simulink model "vehicle_simulation"  (R2020a)
settings: Solver=ode1  StartTime=0.0  StopTime=500  FixedStep=0.1  RelTol=1e-3
undefined symbols (not defined in the file): HDBK, MIL, serial
libraries: powerlib_meascontrol x7, aerolibconvert2 x5, aerolibatmos2 x3, instrumentlib x3, dspsrcs4 x2, simulink x1
(part 5 of 5)

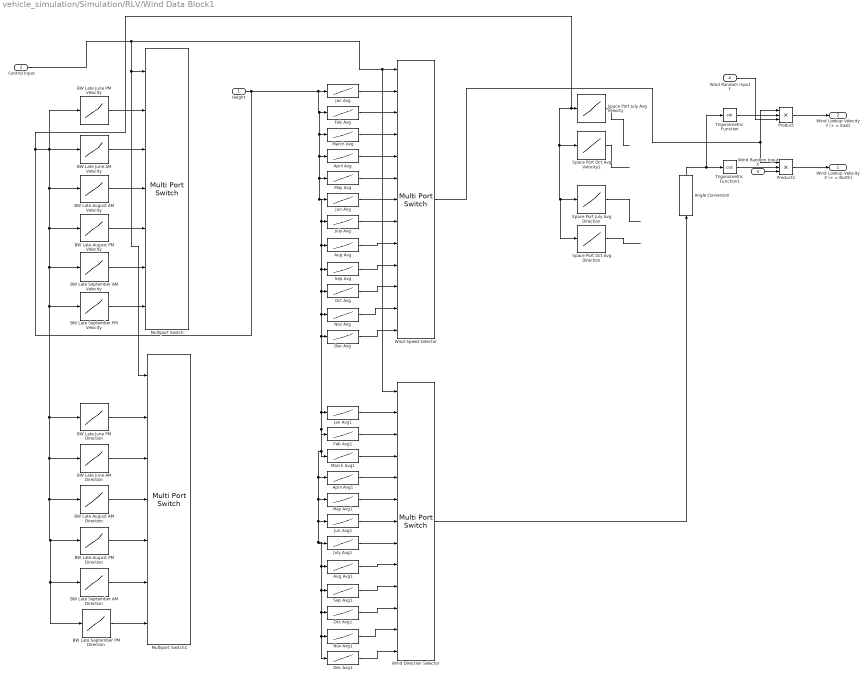
== system vehicle_simulation/Simulation/RLV/Wind Data Block1 ==
  Height : Inport
  Control Input : Inport  Port=2
  Wind Random Input X : Inport  Port=3
  Wind Random Input Y : Inport  Port=4
  Angle Conversion : aerolibconvert2/Angle Conversion  IU=deg  OU=rad
  April Avg : Lookup_n-D  NumberOfTableDimensions=1  BreakpointsForDimension1=[0,5000,10000,15000,20000,24000,100000]  Table=[5,17,30,20,5,7,0]  ExtrapMethod=Clip  UseLastTableValue=on  InternalRulePriority=Speed  RndMeth=Simplest  InputSameDT=on
  April Avg1 : Lookup_n-D  NumberOfTableDimensions=1  BreakpointsForDimension1=[0,5000,10000,15000,20000,24000,100000]  Table=[76,81,82,78,76,69,69]  ExtrapMethod=Clip  UseLastTableValue=on  InternalRulePriority=Speed  RndMeth=Simplest  InputSameDT=on
  Aug Avg : Lookup_n-D  NumberOfTableDimensions=1  BreakpointsForDimension1=[0,5000,10000,15000,20000,24000,100000]  Table=[2,2,5,2,10,14,0]  ExtrapMethod=Clip  UseLastTableValue=on  InternalRulePriority=Speed  RndMeth=Simplest  InputSameDT=on
  Aug Avg1 : Lookup_n-D  NumberOfTableDimensions=1  BreakpointsForDimension1=[0,5000,10000,15000,20000,24000,100000]  Table=[4,289,63,315,273,275,275]  ExtrapMethod=Clip  UseLastTableValue=on  InternalRulePriority=Speed  RndMeth=Simplest  InputSameDT=on
  BW Late August AM Direction : Lookup_n-D  NumberOfTableDimensions=1  BreakpointsForDimension1=[1546.1,1672.3,1845.1,2022.5,2255.5,2513.3,2836.4,3141.1,3395.8,3721.8,4061.2,4331.2,4582.8,4769.4,4942.4,5153.1,5313.9,5529.6,5694.8,5886,6078.5,6266.6,6490.2,6681.6,6882.9,7107.7,7346.2,7560,7827.5,8089.4,8305.8,8552.6,8781.9,9076.5,9311.2,9617.9,9889.3,10128,10375.7,10665.3,10948,11296.3,11552.9,11850.8,12069.6,12365.4,12654,12923.3,13134.5,13346.7,13598.6,13830.3,14097.1,14348,14557.6,14784.6,15036.1,15280.6,15487.7,15749.3,16059.5,16283.4,16572.3,16811.6,17109.6,17372.4,17652.2,17851.6,18135.9,18444.7,18704.6,19006.8,19282,19550.5,19765,20080.7,20374.9,20691.4,21007,21208.3,21458.2,21730.5,22033.2,22269.7,22494.3,22499.6,22744.1,22960,23248.2,23450.9,23683.3,23936.4,24175.2,24392.6,24677.4,24921.7,25201.5,25500,25741.8,25981.6,26271.3,26550.1,26831.4,27099.6,27393,27493.8,27652.2,27741,28143.9,28217,28571.1,28767.7,28789.4,29086.3,29225.3,29399.3,29535.7,29920.3,30157.2,30251.3,30403.5,30734,31253,31646,31990.8,32148.3,32309,32417,32931,80000]  Table=[228.9,227.3,225.3,226.4,224.6,219.5,200.9,219,197.3,198.5,213.3,200.8,219.3,217.2,216.2,215,216,212.2,213.8,202.9,204.9,206.9,207.4,211,201.6,202.9,203.2,190.7,192,192.7,203.6,214.6,223.4,227,228.2,226.7,230.2,241.2,242.4,241.9,251.7,234.8,248.1,248.6,244.7,243.7,243.3,234.7,234.4,236,240.2,238,236.3,234.7,239.7,245.1,241.5,240.7,230.3,236.6,211.5,220.8,210.5,208.3,223.3,205,206.1,209.8,191.8,183.4,190.1,158.7,159.1,163.5,156.7,140,144.3,142.9,122.3,121.3,108.8,108.5,130.9,107,102,113.1,113.8,116.9,92,86.6,84.1,85.1,92.6,93.3,91.3,89.4,96.4,99,99.1,100.8,102.3,100.7,90.3,90.8,91.3,91.1,91,90.4,92.2,99.1,103.4,131.6,99.6,130.4,92.4,89.2,90.2,88.3,91.8,92.5,80,85.3,87.5,94,94.3,102,102.5,97.5,80,0]  InterpMethod=Cubic spline  ExtrapMethod=Clip  UseLastTableValue=on  InternalRulePriority=Speed  RndMeth=Simplest  InputSameDT=on
  BW Late August AM Velocity : Lookup_n-D  NumberOfTableDimensions=1  BreakpointsForDimension1=[1546.1,1672.3,1845.1,2022.5,2255.5,2513.3,2836.4,3141.1,3395.8,3721.8,4061.2,4331.2,4582.8,4769.4,4942.4,5153.1,5313.9,5529.6,5694.8,5886,6078.5,6266.6,6490.2,6681.6,6882.9,7107.7,7346.2,7560,7827.5,8089.4,8305.8,8552.6,8781.9,9076.5,9311.2,9617.9,9889.3,10128,10375.7,10665.3,10948,11296.3,11552.9,11850.8,12069.6,12365.4,12654,12923.3,13134.5,13346.7,13598.6,13830.3,14097.1,14348,14557.6,14784.6,15036.1,15280.6,15487.7,15749.3,16059.5,16283.4,16572.3,16811.6,17109.6,17372.4,17652.2,17851.6,18135.9,18444.7,18704.6,19006.8,19282,19550.5,19765,20080.7,20374.9,20691.4,21007,21208.3,21458.2,21730.5,22033.2,22269.7,22494.3,22499.6,22744.1,22960,23248.2,23450.9,23683.3,23936.4,24175.2,24392.6,24677.4,24921.7,25201.5,25500,25741.8,25981.6,26271.3,26550.1,26831.4,27099.6,27393,27493.8,27652.2,27741,28143.9,28217,28571.1,28767.7,28789.4,29086.3,29225.3,29399.3,29535.7,29920.3,30157.2,30251.3,30403.5,30734,31253,31646,31990.8,32148.3,32309,32417,32931,40000,200000]  Table=[10.3,11.3,12.2,11.7,10.8,8.9,7.9,7.6,7.1,7.1,7.8,8.5,8.7,9.2,10,11.3,11.8,12.9,14.2,14.7,15.3,15.8,15.9,16.1,16.3,16,16.4,16.6,17.2,17.5,17.9,18.4,19,20.1,21.1,22.7,24.6,25.8,27.4,28.5,28.4,28.4,29.3,30,29.4,29.7,29.4,29.1,28.4,28.2,27.7,26.8,24.5,24,23.5,21.6,21.7,21.1,20,19.1,17.9,18.3,17.7,17.2,13.9,13.8,13.7,13.1,13.3,12.9,13.5,12.3,12.8,12.9,13,11.1,12.9,14.2,14.6,13.8,14.7,14.7,33,13.8,15.5,16.5,15.4,14.9,14.7,15.3,15.9,16.3,18.3,18.1,17.9,19,18.7,18.7,18.1,18.7,18.2,18.5,19,19.3,18.5,19.5,17.7,18,19.9,20.5,20.4,58.3,17.7,75.1,22.6,24.3,28.3,27.8,23.5,30.8,28.3,31,34.5,35,29,25,25.5,25,21,0,0]  ExtrapMethod=Clip  UseLastTableValue=on  InternalRulePriority=Speed  RndMeth=Simplest  InputSameDT=on
  BW Late August PM Direction : Lookup_n-D  NumberOfTableDimensions=1  BreakpointsForDimension1=[1558.5,1648.2,1789.4,1938.7,2151.8,2319.3,2551,2766.5,3025.6,3277.9,3544.8,3755.7,4079.3,4350.8,4619.6,4803.8,4944,5138.8,5319.8,5440.2,5599.4,5838,5997.6,6146.9,6269.3,6497.5,6682.2,6901.2,7131.4,7367.7,7576.6,7763.6,7994.5,8193.5,8495.4,8736.4,9025.3,9286.7,9656.1,9897.6,10213.4,10484.2,10783.5,11119.4,11398.6,11714.5,11996.2,12207.4,12522.6,12785.2,13071.9,13369.2,13669.8,13935,14193,14477.3,14699.3,15070.3,15357.4,15583.1,15796,16047.2,16277,16506.1,16719,17040.2,17328.9,17604.3,17903.8,18186,18516.3,18765.9,19090.8,19373.1,19670.9,19978.1,20261.3,20551.4,20782.3,21001.5,21215.2,21495.2,21807,22024.6,22264.8,22540.7,22848.8,23150.7,23414.7,23678.5,23912.6,24191,24462.2,24715.3,24958,24979.7,25287.7,25531.9,25842.2,26076.9,26379.2,26693.5,26874.9,27076,27373,27628.9,27911.3,28064.2,28377.6,28449.7,28781.9,29085.5,29424,29499.6,29734.4,29898.8,30086.3,30412.6,30573.1,30816.7,31075.6,31391.6,31650.9,31971.8,32103.8,32142.4,32186.9,32416.6,32535.9,32768.1,32932.8,33299.5,33428.5,33731,34063.7,80000]  Table=[245.6,248.8,233.6,224.2,206.7,204.7,170,175.9,150.7,153.4,158.9,171.2,180.4,185.1,188.8,194.5,197.3,202.4,208.7,199.6,202.2,206.1,211.7,210.3,224.9,210.6,229.4,228.9,230.5,242.5,226.4,248.2,247.6,242.3,240.3,240.7,237.7,238.1,223.8,237.2,238.6,239.1,238,252.5,250.7,251.9,253.9,243.4,246.2,246.3,248.5,247.6,248.5,235.9,247.5,237.9,230.6,243.6,231.8,238.6,237.1,233.7,226.7,216.2,211.9,226.1,199.2,194.3,199.3,181.4,192.9,198,189.2,187.5,181.9,149.5,147.8,122.4,107.6,124.3,128.1,120.6,125.8,130.7,132.6,97.2,99.2,101.8,103,102.8,88.2,104,102,102.4,88.4,89.1,79.8,81.2,84.6,92.9,100.3,83.6,83.3,87.8,90,85.8,111.6,85.4,88,82.2,88.3,90.2,83.9,83.5,86.3,85.2,89.5,125.8,89.7,92.7,90.1,85.5,90.4,85.4,86.4,82.5,85.9,89.6,92.3,90.8,96.3,91.7,85,83.3,85,0]  InterpMethod=Cubic spline  ExtrapMethod=Clip  UseLastTableValue=on  InternalRulePriority=Speed  RndMeth=Simplest  InputSameDT=on
  BW Late August PM Velocity : Lookup_n-D  NumberOfTableDimensions=1  BreakpointsForDimension1=[1558.5,1648.2,1789.4,1938.7,2151.8,2319.3,2551,2766.5,3025.6,3277.9,3544.8,3755.7,4079.3,4350.8,4619.6,4803.8,4944,5138.8,5319.8,5440.2,5599.4,5838,5997.6,6146.9,6269.3,6497.5,6682.2,6901.2,7131.4,7367.7,7576.6,7763.6,7994.5,8193.5,8495.4,8736.4,9025.3,9286.7,9656.1,9897.6,10213.4,10484.2,10783.5,11119.4,11398.6,11714.5,11996.2,12207.4,12522.6,12785.2,13071.9,13369.2,13669.8,13935,14193,14477.3,14699.3,15070.3,15357.4,15583.1,15796,16047.2,16277,16506.1,16719,17040.2,17328.9,17604.3,17903.8,18186,18516.3,18765.9,19090.8,19373.1,19670.9,19978.1,20261.3,20551.4,20782.3,21001.5,21215.2,21495.2,21807,22024.6,22264.8,22540.7,22848.8,23150.7,23414.7,23678.5,23912.6,24191,24462.2,24715.3,24958,24979.7,25287.7,25531.9,25842.2,26076.9,26379.2,26693.5,26874.9,27076,27373,27628.9,27911.3,28064.2,28377.6,28449.7,28781.9,29085.5,29424,29499.6,29734.4,29898.8,30086.3,30412.6,30573.1,30816.7,31075.6,31391.6,31650.9,31971.8,32103.8,32142.4,32186.9,32416.6,32535.9,32768.1,32932.8,33299.5,33428.5,33731,34063.7,40000,200000]  Table=[4.8,5.5,6,5.9,7.2,8.1,8.5,9,9.3,10.8,11.7,12.9,14.8,15.7,16.5,16.8,16.9,16.6,15.7,15.8,15.7,15.5,15.2,14.4,15.1,15,15.5,15.1,15,15.3,16.3,16.9,17.6,18.4,19.6,20.3,21.4,22.5,24.1,25.2,26.4,27.7,28.3,29.7,31.1,32,32.5,31.9,31.3,30.1,28.9,29.1,28.9,29.6,29.4,27.7,27.2,27.7,26.3,24.7,23.7,22.4,21.1,21.2,21.7,19.5,16.6,15.3,13.9,14,13.2,12.7,11.7,11.4,11.9,11.2,11.6,13.9,12.9,12.8,14.2,13.6,12.1,12.6,12.7,12.3,12.1,13.9,13.1,14.3,16.4,16.7,17.3,18.4,17.2,16.1,17.6,19,20.5,18.6,17.2,18.4,20,21.5,19.7,19.8,54.9,21.9,22.8,20.5,23.4,22.7,22,25,24.9,25,25.4,68.5,27.5,28,27.6,26.9,26.8,26.1,24.6,30,28.7,29.5,30.2,29.7,29,27.7,28.7,28,20,0,0]  ExtrapMethod=Clip  UseLastTableValue=on  InternalRulePriority=Speed  RndMeth=Simplest  InputSameDT=on
  BW Late June AM Direction : Lookup_n-D  NumberOfTableDimensions=1  BreakpointsForDimension1=[1536,1649.9,1826.3,1987.3,2223.7,2471.2,2753.2,3051.3,3313.6,3561.6,3761.2,3963.1,4153.1,4376.3,4528.3,4732.8,4902.4,5114.1,5270.8,5523.3,5743.3,5961.6,6179.3,6469.3,6758.8,7028.7,7197,7498.4,7737.9,8019,8232.9,8512.3,8841.8,9135.1,9445.3,9739.9,10023,10371.1,10692.7,10974.1,11288.3,11517.6,11773.9,12093,12308.2,12547.9,12782.4,13043.9,13311.8,13522.3,13743.5,13949.8,14153.6,14382.6,14607.5,14815.1,15045.4,15265.9,15492.9,15685.5,15913.4,16155.2,16378.7,16669.4,16925.3,17164.9,17385.2,17681,17939.9,18210.3,18517.3,18733.7,18940,19233.6,19478.7,19748.2,19966.6,20259.7,20584.8,20834.6,21150.2,21428.3,21702.8,21984.6,22266.5,22580.8,22910.6,23197.4,23405.3,23664.9,23970.1,24306,24608.9,24854.4,25152.9,25385.6,25732.1,26039.1,26287,26528.2,26810.2,27136.8,27443,27862.2,28053.3,28427.7,28698.3,29149.1,29466,29647.1,29819.8,30150.6,30284.6,30388.1,30808.2,31027,31391.5,31520,31699,31875]  Table=[236.7,234.9,219.7,243.9,231.7,235.3,236,250,250,244.1,246.1,241.1,243.4,234.3,232.3,242.3,242.1,241.7,242.3,241.9,243.3,245.3,246.3,252.4,255.9,246.8,246.6,234.8,234.3,235.2,234.1,233.6,247.6,249.8,248.2,257.9,257.3,257.4,258.2,257.7,258.4,247.7,259.2,259.7,259.9,261.8,261.3,260.5,261.4,263.1,258,257.4,257,256.7,258.7,260.7,264.1,255.3,256.3,257.4,258.7,253.1,249.1,225.8,224,203,201,194.1,209.9,191,190.5,181.4,167.8,161.1,154.4,152.3,145.2,154.2,160.1,161,154.5,151.8,119.6,116.3,132.7,137.5,114.3,113,109.1,113.9,119.5,136.3,109.3,104.1,104.8,85.9,104.8,90.1,91.3,96.8,101.7,105.7,111.1,97,106.5,110.7,104.1,83.8,92.3,97,97.2,101.7,99.6,90.6,91.5,87.3,80,155,110,110]  InterpMethod=Cubic spline  ExtrapMethod=Clip  UseLastTableValue=on  InternalRulePriority=Speed  RndMeth=Simplest  InputSameDT=on
  BW Late June AM Velocity : Lookup_n-D  NumberOfTableDimensions=1  BreakpointsForDimension1=[1536,1649.9,1826.3,1987.3,2223.7,2471.2,2753.2,3051.3,3313.6,3561.6,3761.2,3963.1,4153.1,4376.3,4528.3,4732.8,4902.4,5114.1,5270.8,5523.3,5743.3,5961.6,6179.3,6469.3,6758.8,7028.7,7197,7498.4,7737.9,8019,8232.9,8512.3,8841.8,9135.1,9445.3,9739.9,10023,10371.1,10692.7,10974.1,11288.3,11517.6,11773.9,12093,12308.2,12547.9,12782.4,13043.9,13311.8,13522.3,13743.5,13949.8,14153.6,14382.6,14607.5,14815.1,15045.4,15265.9,15492.9,15685.5,15913.4,16155.2,16378.7,16669.4,16925.3,17164.9,17385.2,17681,17939.9,18210.3,18517.3,18733.7,18940,19233.6,19478.7,19748.2,19966.6,20259.7,20584.8,20834.6,21150.2,21428.3,21702.8,21984.6,22266.5,22580.8,22910.6,23197.4,23405.3,23664.9,23970.1,24306,24608.9,24854.4,25152.9,25385.6,25732.1,26039.1,26287,26528.2,26810.2,27136.8,27443,27862.2,28053.3,28427.7,28698.3,29149.1,29466,29647.1,29819.8,30150.6,30284.6,30388.1,30808.2,31391.5,31520,31699,31875,40000,200000]  Table=[12,12.7,13.9,13.8,13.2,13.2,13,13.6,13.5,13.8,14.7,15.9,17.7,18.8,20.3,21.1,21.1,21.9,22.3,23.3,24.2,24.4,25.5,26.4,27.5,29.7,30.6,32.9,34.3,35.9,36.6,36.8,37.6,38.6,40.4,42,42.8,43.6,45.2,45.8,44.4,44.2,44.9,45,44.5,44.5,44.7,44.7,44.9,43.7,42.2,40,39.3,37.7,35.8,35.3,33.7,31.8,30.9,28.8,26.1,24.7,23.1,20.8,19.7,18.8,18.8,17.8,17,16.2,14.7,13.4,14.1,14,13.9,13.2,12.9,12.8,12.9,11.8,10.8,10.8,11.4,11.8,11.3,11.1,11.3,11.9,12.7,13.3,11.9,12.2,11.8,13,13,13.8,14,13.9,13.7,15.3,14.8,14.3,14.2,14.3,14.9,14.3,13,11.7,12.5,14.6,16.4,16,15.2,16,19.2,23,10,7,0,0,0]  ExtrapMethod=Clip  UseLastTableValue=on  InternalRulePriority=Speed  RndMeth=Simplest  InputSameDT=on
  BW Late June PM Direction : Lookup_n-D  NumberOfTableDimensions=1  BreakpointsForDimension1=[1539.6,1647.8,1799.9,1942.5,2137.8,2321.9,2532.1,2706.3,2902.8,3066.6,3234,3421.5,3544.4,3690.8,3880.5,4076.9,4198.9,4396.9,4604.2,4817.8,5047.1,5277.1,5497.6,5710.4,5916.2,6144.4,6351.4,6584.6,6807.2,7032.3,7274.6,7543.6,7758.9,7945.6,8170.1,8502.2,8676.3,8954.7,9194,9436.2,9680.7,9976.7,10223.6,10484.4,10728.5,11092.4,11314.9,11546.3,11877.1,12134.6,12397.9,12662.9,12940.1,13185.5,13494.8,13757.4,14005,14311.4,14520.4,14761.3,14956.1,15161.4,15378.9,15614.6,15844.3,16068.3,16285.6,16527.2,16789.7,17077.7,17299.8,17583.4,17856.4,18103.7,18393.9,18643.3,18917.1,19155,19510.1,19770.5,20085.9,20364.4,20581.1,20835.4,21070.6,21327.9,21629.5,21884.1,22140.7,22466.9,22743.1,23012.4,23258.6,23582.5,23892.5,24149.5,24500.6,24774.7,25107.4,25323.1,25570,25845.4,26138.5,26438.1,27090.5,27336.6,27664.1,27969.9,28239.2,28559.2,28627.6,28766.6,28965.5,29363.6,29633.1,29782.6,29952.7,29994.2,30286,30636.8,30912.1,31243.4,31300.1,31641.7,31947.6,32125.4,32745.7,33053,33161]  Table=[202.7,219.4,216.1,215.6,209.4,189.1,197.3,191.7,201.2,202.4,199.1,202.2,207.2,213.8,215.6,218.2,220.9,225.4,225.6,235.2,235.4,235.7,237.4,238.4,238.5,238.4,236.8,238.5,238.8,240,239.6,250.6,250,248.6,247.1,248.3,249.9,249.5,249.3,249.7,252.8,255.9,254,254,253.3,255.2,257,257.4,257.6,256.3,256,255.4,255.6,256.5,257.9,258.8,258.3,244.8,245.9,249.7,250.5,240.3,231.2,249.2,250.3,249.5,250.4,231.7,221.9,202.2,213.8,200.5,201.8,213.6,190,187.3,179.4,168.8,176,166.7,146.2,155.1,145.3,140.3,132.7,132.8,122.3,135.3,127.2,121.9,119.2,121.9,114.9,92.2,100.8,105.1,103.1,102.6,96.1,101.1,84.9,89.4,103.9,99.1,104.3,89.1,78.7,82.9,73.2,72,90,85.7,86.6,87.1,95.1,86.9,93.8,101.5,94.8,100.8,89.8,90.7,127.5,106.8,95.3,95.2,93.5,93,90]  InterpMethod=Cubic spline  ExtrapMethod=Clip  UseLastTableValue=on  InternalRulePriority=Speed  RndMeth=Simplest  InputSameDT=on
  BW Late June PM Velocity : Lookup_n-D  NumberOfTableDimensions=1  BreakpointsForDimension1=[1539.6,1647.8,1799.9,1942.5,2137.8,2321.9,2532.1,2706.3,2902.8,3066.6,3234,3421.5,3544.4,3690.8,3880.5,4076.9,4198.9,4396.9,4604.2,4817.8,5047.1,5277.1,5497.6,5710.4,5916.2,6144.4,6351.4,6584.6,6807.2,7032.3,7274.6,7543.6,7758.9,7945.6,8170.1,8502.2,8676.3,8954.7,9194,9436.2,9680.7,9976.7,10223.6,10484.4,10728.5,11092.4,11314.9,11546.3,11877.1,12134.6,12397.9,12662.9,12940.1,13185.5,13494.8,13757.4,14005,14311.4,14520.4,14761.3,14956.1,15161.4,15378.9,15614.6,15844.3,16068.3,16285.6,16527.2,16789.7,17077.7,17299.8,17583.4,17856.4,18103.7,18393.9,18643.3,18917.1,19155,19510.1,19770.5,20085.9,20364.4,20581.1,20835.4,21070.6,21327.9,21629.5,21884.1,22140.7,22466.9,22743.1,23012.4,23258.6,23582.5,23892.5,24149.5,24500.6,24774.7,25107.4,25323.1,25570,25845.4,26138.5,26438.1,26773.1,27090.5,27336.6,27664.1,27969.9,28239.2,28559.2,28627.6,28766.6,28965.5,29363.6,29633.1,29782.6,29952.7,29994.2,30286,30636.8,30912.1,31243.4,31300.1,31641.7,31947.6,32125.4,32745.7,33053,33161,40000,200000]  Table=[6,6.7,7.1,8,8.8,9.8,10.4,11.3,12,13.4,14.7,16.3,16.9,18.1,18.9,19.5,19.7,21,21.9,22.6,24.2,25.3,26,26.3,27.3,27.9,28.8,29.4,30.3,31.3,33.1,35,35.9,36,36.4,37,37.5,38,38.9,39.6,41.7,42.8,43.4,45.7,47.6,48.4,50.5,52,52,52.1,52,51.1,50.4,50.2,48.3,46.9,44.2,43,42.4,40.5,38.4,37.1,36.9,34.6,32.3,30.4,28.6,27.8,24.5,21.1,20.1,19.3,19.7,19.3,17.9,16.9,16.1,15.3,14,14,14,12.7,11.7,11.6,10.8,11.8,11.9,11.5,12.3,12.8,11.9,11.8,13.2,13,12.3,10.7,13.6,14.8,16,16.6,15.1,14.2,13.7,13.8,15.5,14.3,14.4,14.6,15.2,14.5,14.7,16.2,16.1,16.8,16,15.9,16.7,17.4,17.4,19.2,20.4,20.5,21.5,19.2,20.2,21.5,22.7,35,23,10,0,0]  ExtrapMethod=Clip  UseLastTableValue=on  InternalRulePriority=Speed  RndMeth=Simplest  InputSameDT=on
  BW Late September AM Direction : Lookup_n-D  NumberOfTableDimensions=1  BreakpointsForDimension1=[1546,1668.7,1841.7,2045.9,2293.6,2534.9,2799.3,3077.5,3304.1,3475.9,3698.9,3881.6,4072.5,4220.2,4414.3,4576.6,4724.1,4918.7,5124,5324.5,5574.7,5743.7,5985.4,6220.2,6402.4,6639,6821.4,7039.9,7230.9,7548.5,7732.1,7888,8102.2,8304.5,8579.2,8800.9,9085.2,9354.5,9685.1,9920.9,10116.9,10439.8,10683.1,10956.9,11143.9,11361.3,11604,11871.7,12042.4,12261.1,12514,12729.1,12924.4,13134.4,13335.7,13567.9,13743.1,13972.6,14201.4,14435.9,14670.3,14985,15226,15547.6,15775.1,16073.5,16296.4,16582.9,16919.6,17200.8,17426.3,17743.3,17977.4,18296,18608.2,18884.1,19177.6,19427.6,19642.6,19912.7,20235.6,20534.6,20794.6,21164.5,21409.9,21737.5,22060.2,22392.7,22651.1,22943.4,23235.4,23534.3,23921.9,24225.6,24474.9,24835.1,25150.3,25518.8,25804.6,26045.4,26217.5,26519.6,26777.4,27081.2,27340.1,27614.3,27724.8,27903.6,28253.8,28471.2,28796.3,29023.3,29121.5,29150.3,29210.9,29271.3,29470,29819.1,30151.3,30597.6,30944.4,32044.5,32087.7,32319.3,32716,32920.3,33151,33369,33833,33920,34073.5,34442]  Table=[164.2,164.2,162.8,159.9,156.1,182,186,181,165.8,176.2,174.5,170.9,179.4,181.3,177.6,181.1,181.3,178.5,180.8,184,187.8,188.4,188.6,176.7,190.9,189.5,188.9,190.8,180.1,205.1,206,206.7,205.1,208,210.1,210.7,225,225.7,212.1,212,211.7,211.3,209,208,219.5,219.7,230.7,231.2,217.6,207.4,210.3,224.5,237,237.6,238.2,239.2,242.2,234.1,224,220.3,227.7,232.5,217.7,218.9,210.6,216.4,220.1,217.6,216.2,229.7,223.4,201.2,191,202.2,202.8,200,180,182.3,175.3,193.4,199.6,182.5,177,141,146.5,136.4,145.4,148.3,159.6,169,168.1,159.4,177.7,142,129.9,140.4,146.4,164.9,169.9,169.4,186.8,182.5,159.7,191,198.3,186.5,158.3,148.4,150.9,148.8,153.9,137,99.5,87.5,192.8,179,108.2,122.4,126,123,112.1,187,68,101.3,58.3,105,101.5,137.5,227.5,243,275,245]  InterpMethod=Cubic spline  ExtrapMethod=Clip  UseLastTableValue=on  InternalRulePriority=Speed  RndMeth=Simplest  InputSameDT=on
  BW Late September AM Velocity : Lookup_n-D  NumberOfTableDimensions=1  BreakpointsForDimension1=[1546,1668.7,1841.7,2045.9,2293.6,2534.9,2799.3,3077.5,3304.1,3475.9,3698.9,3881.6,4072.5,4220.2,4414.3,4576.6,4724.1,4918.7,5124,5324.5,5574.7,5743.7,5985.4,6220.2,6402.4,6639,6821.4,7039.9,7230.9,7548.5,7732.1,7888,8102.2,8304.5,8579.2,8800.9,9085.2,9354.5,9685.1,9920.9,10116.9,10439.8,10683.1,10956.9,11143.9,11361.3,11604,11871.7,12042.4,12261.1,12514,12729.1,12924.4,13134.4,13335.7,13567.9,13743.1,13972.6,14201.4,14435.9,14670.3,14985,15226,15547.6,15775.1,16073.5,16296.4,16582.9,16919.6,17200.8,17426.3,17743.3,17977.4,18296,18608.2,18884.1,19177.6,19427.6,19642.6,19912.7,20235.6,20534.6,20794.6,21164.5,21409.9,21737.5,22060.2,22392.7,22651.1,22943.4,23235.4,23534.3,23921.9,24225.6,24474.9,24835.1,25150.3,25518.8,25804.6,26045.4,26217.5,26519.6,26777.4,27081.2,27340.1,27614.3,27724.8,27903.6,28253.8,28471.2,28796.3,28996.3,29121.5,29150.3,29210.9,29271.3,29470,29819.1,30151.3,30597.6,30883.3,31717.3,32087.7,32319.3,32716,32920.3,33151,33369,33833,33920,34073.5,34442,40000,200000]  Table=[11.5,12.4,13.9,14.2,13.7,13.2,13.4,13.5,13.6,13.9,14.8,15.8,16.2,17.4,19.2,20.5,21.3,22.8,23.2,22.9,23.3,23.7,24.9,26.1,27,27.6,28.4,30.2,30.5,31.6,32.6,33.4,35.1,36,36.4,37.3,38,38.6,38.8,39.8,40.6,41.4,41.6,41.7,42.1,42.7,42.8,41.6,39.7,39.3,38.7,38,37.3,36,34.1,31.8,30.1,28.8,27.6,27.1,26.3,24.6,23.8,23.4,21.2,19.8,18.9,18.9,17.2,16.7,17.3,16.9,14.7,13.6,13.6,12.6,12.6,12.3,11.3,11,11.7,11.5,9.9,11.7,12.2,11.7,11.9,11.8,11.7,10.5,10.5,10.7,12.5,13.2,11.9,12.3,11.6,11.8,11.1,11.8,11.3,10.2,10.6,10.9,11.2,9,11.4,12.6,11.5,12.1,9.3,10.9,8.8,8.2,10.9,12,10.6,10.2,12.6,13.8,11.5,9.3,12.7,15.3,14.7,7.7,14.5,15.5,10,9,9,14,0,0]  ExtrapMethod=Clip  UseLastTableValue=on  InternalRulePriority=Speed  RndMeth=Simplest  InputSameDT=on
  BW Late September PM Direction : Lookup_n-D  NumberOfTableDimensions=1  BreakpointsForDimension1=[1527.8,1631.8,1792.4,1937.7,2135.6,2342.5,2541.7,2762.7,2984.3,3166.7,3404.2,3589.1,3756.1,3951.2,4156.9,4327.9,4516.6,4663,4820.6,5006.7,5219.7,5397.8,5561,5779.9,5946.5,6163.8,6354.9,6563.2,6759.4,6942.2,7147.1,7404.2,7606,7847.9,8126.1,8334.2,8619.4,8904.6,9146.3,9335.6,9568.6,9837.6,10034.8,10233,10482.5,10781.7,10989.5,11194.8,11404.6,11663.2,11882.9,12133.7,12304.6,12537.4,12786.7,13072.9,13320.1,13473.6,13719.8,13973.2,14196.5,14474.5,14729.9,14953.6,15195.7,15433.5,15630,15844.7,16064,16372,16645.5,16917.5,17204.8,17475.5,17733,17969.4,18275,18586.1,18883.8,19156.6,19390.5,19629.3,19881.3,20146.7,20559,20901.6,21234.5,21533.3,21803.9,22100.5,22454.2,22776.8,23106,23405.3,23721.9,24043.9,24366.5,24781.4,25175.9,25482.6,25853.3,26189.5,26560.5,26949,27318.8,27671.8,27943.7,28195.6,28238.2,28620.5,28944.9,29226,29271.1,29536.8,29894,30128.6,30377.8,30455.8,30588.9,30709.3,30788.4,30923,31190.9,31409.8,31756.4,32048,32436.7,32614.1,33073.4,33235.5,33482,33579,33929,34330,34999,35239,35662,36020,36271,36445,80000]  Table=[179.8,213.7,201.4,204.7,151.1,150.4,160.2,166.2,167.9,169.2,171.7,171.8,176,181.9,191.6,189.4,175.6,175.6,177.3,189.6,192.1,204.4,203.7,203.1,203,203.8,205.8,207.5,206.9,218,216.1,215.4,216.5,229.1,217.7,218.9,219.1,244.9,219.4,204.7,208.7,210.1,197.7,209.7,220.3,220.2,219.8,210.2,222.9,234.1,233.2,243.8,245.7,236.7,236.3,223.1,220.8,219.1,217.4,218.2,227.4,223.7,233.7,233.4,228.6,233,222.3,224,223.7,207.8,220.6,220.3,232.1,233.6,242.9,232.5,220.2,197.8,170.3,184.6,175,177.3,173.3,173.9,156.4,173,189.6,190,170.3,156.5,117.5,122.2,155.1,133.3,123.3,124.6,117,107.1,105.1,137.4,159.8,150.6,145.7,143,139.8,128.1,142.3,157.6,143,138.1,155.9,142.8,165.3,164.3,152.3,151.3,169,173.2,143,162.7,189.6,127.1,86.3,181.1,102,108.9,116.4,117,66.5,98.8,137,142.5,100,52,327,328,345,345,50,50,50]  InterpMethod=Cubic spline  ExtrapMethod=Clip  UseLastTableValue=on  InternalRulePriority=Speed  RndMeth=Simplest  InputSameDT=on
  BW Late September PM Velocity : Lookup_n-D  NumberOfTableDimensions=1  BreakpointsForDimension1=[1527.8,1631.8,1792.4,1937.7,2135.6,2342.5,2541.7,2762.7,2984.3,3166.7,3404.2,3589.1,3756.1,3951.2,4156.9,4327.9,4516.6,4663,4820.6,5006.7,5219.7,5397.8,5561,5779.9,5946.5,6163.8,6354.9,6563.2,6759.4,6942.2,7147.1,7404.2,7606,7847.9,8126.1,8334.2,8619.4,8904.6,9146.3,9335.6,9568.6,9837.6,10034.8,10233,10482.5,10781.7,10989.5,11194.8,11404.6,11663.2,11882.9,12133.7,12304.6,12537.4,12786.7,13072.9,13320.1,13473.6,13719.8,13973.2,14196.5,14474.5,14729.9,14953.6,15195.7,15433.5,15630,15844.7,16064,16372,16645.5,16917.5,17204.8,17475.5,17733,17969.4,18275,18586.1,18883.8,19156.6,19390.5,19629.3,19881.3,20146.7,20559,20901.6,21234.5,21533.3,21803.9,22100.5,22454.2,22776.8,23106,23405.3,23721.9,24043.9,24366.5,24781.4,25175.9,25482.6,25853.3,26189.5,26560.5,26949,27318.8,27671.8,27943.7,28195.6,28238.2,28620.5,28944.9,29226,29271.1,29536.8,29894,30128.6,30377.8,30455.8,30588.9,30709.3,30788.4,31190.9,31409.8,31756.4,32048,32436.7,32614.1,33073.4,33235.5,33365.3,33482,33579,33929,34029.5,34330,35052,35239,35662,36020,36271,36445,40000,200000]  Table=[4.7,5.5,7.4,8,9.3,10.5,11,11.7,12.6,13.7,14.9,16.8,18.1,19.4,20.3,21.2,22.4,22.7,23.2,23.6,24,25.2,26,26.8,27.4,27.5,28.6,29.7,31.6,33.2,34.7,37,38.3,38.4,39.6,39.7,40.2,40.5,41.5,41.6,42.2,42.9,44.2,45,44.8,44.7,4.3,44.7,44.4,44.4,43.6,43.9,43.2,42.4,41.6,39.9,39.4,38.7,36.3,35.1,32.6,30,28.3,27.5,26.9,26,25.2,3.8,22.9,22.3,20.5,18.8,17.7,18,17.7,15.8,14.8,14.1,14.3,14.4,14.6,13.9,14.6,13.9,12.3,13.4,12.3,10.5,9.8,9,9.8,10.1,10.5,11,10.4,9.3,10.6,9.6,8.4,9.6,9.5,9,9.5,8.2,8.1,9.8,10.7,9.7,10.5,11.1,11.3,13,12,11.2,10.3,10.2,10.4,11.6,11.9,11.3,12.4,13.8,12.4,17.1,15.4,10.6,11.6,13.2,12.5,9.7,17.5,14,10,11,7,1,7,19,26,10,0,0,0]  ExtrapMethod=Clip  UseLastTableValue=on  InternalRulePriority=Speed  RndMeth=Simplest  InputSameDT=on
  Dec Avg : Lookup_n-D  NumberOfTableDimensions=1  BreakpointsForDimension1=[0,5000,10000,15000,20000,24000,100000]  Table=[2,17,30,23,7,5,0]  ExtrapMethod=Clip  UseLastTableValue=on  InternalRulePriority=Speed  RndMeth=Simplest  InputSameDT=on
  Dec Avg1 : Lookup_n-D  NumberOfTableDimensions=1  BreakpointsForDimension1=[0,5000,10000,15000,20000,24000,100000]  Table=[63,82,86,86,85,83,83]  ExtrapMethod=Clip  UseLastTableValue=on  InternalRulePriority=Speed  RndMeth=Simplest  InputSameDT=on
  Feb Avg : Lookup_n-D  NumberOfTableDimensions=1  BreakpointsForDimension1=[0,5000,10000,15000,20000,24000,100000]  Table=[2,17,30,23,5,2,0]  ExtrapMethod=Clip  UseLastTableValue=on  InternalRulePriority=Speed  RndMeth=Simplest  InputSameDT=on
  Feb Avg1 : Lookup_n-D  NumberOfTableDimensions=1  BreakpointsForDimension1=[0,5000,10000,15000,20000,24000,100000]  Table=[63,88,86,85,83,72,72]  ExtrapMethod=Clip  UseLastTableValue=on  InternalRulePriority=Speed  RndMeth=Simplest  InputSameDT=on
  Jan Avg : Lookup_n-D  NumberOfTableDimensions=1  BreakpointsForDimension1=[0,5000,10000,15000,20000,24000,100000]  Table=[2,17,30,22,5,2,0]  ExtrapMethod=Clip  UseLastTableValue=on  InternalRulePriority=Speed  RndMeth=Simplest  InputSameDT=on
  Jan Avg1 : Lookup_n-D  NumberOfTableDimensions=1  BreakpointsForDimension1=[0,5000,10000,15000,20000,24000,100000]  Table=[63,92,87,86,97,108,108]  ExtrapMethod=Clip  UseLastTableValue=on  InternalRulePriority=Speed  RndMeth=Simplest  InputSameDT=on
  July Avg : Lookup_n-D  NumberOfTableDimensions=1  BreakpointsForDimension1=[0,5000,10000,15000,20000,24000,100000]  Table=[3,2,2,2,10,14,0]  ExtrapMethod=Clip  UseLastTableValue=on  InternalRulePriority=Speed  RndMeth=Simplest  InputSameDT=on
  July Avg1 : Lookup_n-D  NumberOfTableDimensions=1  BreakpointsForDimension1=[0,5000,10000,15000,20000,24000,100000]  Table=[4,263,90,304,273,275,275]  ExtrapMethod=Clip  UseLastTableValue=on  InternalRulePriority=Speed  RndMeth=Simplest  InputSameDT=on
  Jun Avg : Lookup_n-D  NumberOfTableDimensions=1  BreakpointsForDimension1=[0,5000,10000,15000,20000,24000,100000]  Table=[2,5,15,7,7,10,0]  ExtrapMethod=Clip  UseLastTableValue=on  InternalRulePriority=Speed  RndMeth=Simplest  InputSameDT=on
  Jun Avg1 : Lookup_n-D  NumberOfTableDimensions=1  BreakpointsForDimension1=[0,5000,10000,15000,20000,24000,100000]  Table=[53,63,72,59,279,277,277]  ExtrapMethod=Clip  UseLastTableValue=on  InternalRulePriority=Speed  RndMeth=Simplest  InputSameDT=on
  March Avg : Lookup_n-D  NumberOfTableDimensions=1  BreakpointsForDimension1=[0,5000,10000,15000,20000,24000,100000]  Table=[3,17,30,23,5,5,0]  ExtrapMethod=Clip  UseLastTableValue=on  InternalRulePriority=Speed  RndMeth=Simplest  InputSameDT=on
  March Avg1 : Lookup_n-D  NumberOfTableDimensions=1  BreakpointsForDimension1=[0,5000,10000,15000,20000,24000,100000]  Table=[72,87,86,83,76,63,63]  ExtrapMethod=Clip  UseLastTableValue=on  InternalRulePriority=Speed  RndMeth=Simplest  InputSameDT=on
  May Avg : Lookup_n-D  NumberOfTableDimensions=1  BreakpointsForDimension1=[0,5000,10000,15000,20000,24000,100000]  Table=[3,10,20,12,2,2,0]  ExtrapMethod=Clip  UseLastTableValue=on  InternalRulePriority=Speed  RndMeth=Simplest  InputSameDT=on
  May Avg1 : Lookup_n-D  NumberOfTableDimensions=1  BreakpointsForDimension1=[0,5000,10000,15000,20000,24000,100000]  Table=[63,68,79,76,56,63,63]  ExtrapMethod=Clip  UseLastTableValue=on  InternalRulePriority=Speed  RndMeth=Simplest  InputSameDT=on
  Multiport Switch : MultiPortSwitch  Inputs=6
  Multiport Switch1 : MultiPortSwitch  Inputs=6
  Nov Avg : Lookup_n-D  NumberOfTableDimensions=1  BreakpointsForDimension1=[0,5000,10000,15000,20000,24000,100000]  Table=[2,12,30,20,7,7,0]  ExtrapMethod=Clip  UseLastTableValue=on  InternalRulePriority=Speed  RndMeth=Simplest  InputSameDT=on
  Nov Avg1 : Lookup_n-D  NumberOfTableDimensions=1  BreakpointsForDimension1=[0,5000,10000,15000,20000,24000,100000]  Table=[63,89,87,85,78,58,58]  ExtrapMethod=Clip  UseLastTableValue=on  InternalRulePriority=Speed  RndMeth=Simplest  InputSameDT=on
  Oct Avg : Lookup_n-D  NumberOfTableDimensions=1  BreakpointsForDimension1=[0,5000,10000,15000,20000,24000,100000]  Table=[2,10,23,12,5,2,0]  ExtrapMethod=Clip  UseLastTableValue=on  InternalRulePriority=Speed  RndMeth=Simplest  InputSameDT=on
  Oct Avg1 : Lookup_n-D  NumberOfTableDimensions=1  BreakpointsForDimension1=[0,5000,10000,15000,20000,24000,100000]  Table=[27,79,81,80,76,45,45]  ExtrapMethod=Clip  UseLastTableValue=on  InternalRulePriority=Speed  RndMeth=Simplest  InputSameDT=on
  Product : Product  Inputs=3
  Product1 : Product  Inputs=3
  Sep Avg : Lookup_n-D  NumberOfTableDimensions=1  BreakpointsForDimension1=[0,5000,10000,15000,20000,24000,100000]  Table=[2,5,17,7,5,7,0]  ExtrapMethod=Clip  UseLastTableValue=on  InternalRulePriority=Speed  RndMeth=Simplest  InputSameDT=on
  Sep Avg1 : Lookup_n-D  NumberOfTableDimensions=1  BreakpointsForDimension1=[0,5000,10000,15000,20000,24000,100000]  Table=[27,73,79,76,277,281,281]  ExtrapMethod=Clip  UseLastTableValue=on  InternalRulePriority=Speed  RndMeth=Simplest  InputSameDT=on
  Space Port July Avg Direction : Lookup_n-D  NumberOfTableDimensions=1  BreakpointsForDimension1=[0,5000,10000,15000,20000,25000,30000,200000]  Table=[175,140,175,140,100,80,80,80]  ExtrapMethod=Clip  UseLastTableValue=on  InternalRulePriority=Speed  RndMeth=Simplest  InputSameDT=on
  Space Port July Avg Velocity : Lookup_n-D  NumberOfTableDimensions=1  BreakpointsForDimension1=[0,5000,10000,15000,20000,25000,30000,200000]  Table=[10,15,18,19,19,25,35,0]  ExtrapMethod=Clip  UseLastTableValue=on  InternalRulePriority=Speed  RndMeth=Simplest  InputSameDT=on
  Space Port Oct Avg Direction : Lookup_n-D  NumberOfTableDimensions=1  BreakpointsForDimension1=[0,5000,10000,15000,20000,25000,30000,200000]  Table=[180,230,260,250,200,140,140,140]  ExtrapMethod=Clip  UseLastTableValue=on  InternalRulePriority=Speed  RndMeth=Simplest  InputSameDT=on
  Space Port Oct Avg Velocity1 : Lookup_n-D  NumberOfTableDimensions=1  BreakpointsForDimension1=[0,5000,10000,15000,20000,25000,30000,200000]  Table=[10,18,40,35,15,15,20,0]  ExtrapMethod=Clip  UseLastTableValue=on  InternalRulePriority=Speed  RndMeth=Simplest  InputSameDT=on
  Trigonometric Function : Trigonometry
  Trigonometric Function1 : Trigonometry  Operator=cos
  Wind Direction Selector : MultiPortSwitch  Inputs=12
  Wind Speed Selector : MultiPortSwitch  Inputs=12
  Wind Lookup Velocity X (+ = North) : Outport  VectorParamsAs1DForOutWhenUnconnected=off
  Wind Lookup Velocity Y (+ = East) : Outport  Port=2  VectorParamsAs1DForOutWhenUnconnected=off
  wires:
  Trigonometric Function/1 -> Product/2
  Trigonometric Function1/1 -> Product1/2
  Product1/1 -> Wind Lookup Velocity X (+ = North)/1
  Product/1 -> Wind Lookup Velocity Y (+ = East)/1
  BW Late June PM Velocity/1 -> Multiport Switch/2
  BW Late June PM Direction/1 -> Multiport Switch1/2
  Angle Conversion/1 -> Trigonometric Function1/1, Trigonometric Function/1
  BW Late June AM Velocity/1 -> Multiport Switch/3
  BW Late August AM Velocity/1 -> Multiport Switch/4
  BW Late August PM Velocity/1 -> Multiport Switch/5
  BW Late September AM Velocity/1 -> Multiport Switch/6
  BW Late September PM Velocity/1 -> Multiport Switch/7
  Height/1 -> Dec Avg1/1, Nov Avg1/1, Oct Avg1/1, Sep Avg1/1, Aug Avg1/1, July Avg1/1, Jun Avg1/1, May Avg1/1, April Avg1/1, March Avg1/1, Feb Avg1/1, Jan Avg1/1, Dec Avg/1, Nov Avg/1, Oct Avg/1, Sep Avg/1, Aug Avg/1, July Avg/1, Jun Avg/1, May Avg/1, April Avg/1, March Avg/1, Feb Avg/1, Jan Avg/1, Space Port Oct Avg Velocity1/1, Space Port Oct Avg Direction/1, Space Port July Avg Direction/1, Space Port July Avg Velocity/1, BW Late June AM Velocity/1, BW Late August AM Velocity/1, BW Late August PM Velocity/1, BW Late September PM Direction/1, BW Late September AM Direction/1, BW Late August PM Direction/1, BW Late August AM Direction/1, BW Late June AM Direction/1, BW Late June PM Direction/1, BW Late September PM Velocity/1, BW Late September AM Velocity/1, BW Late June PM Velocity/1
  BW Late June AM Direction/1 -> Multiport Switch1/3
  BW Late August AM Direction/1 -> Multiport Switch1/4
  BW Late August PM Direction/1 -> Multiport Switch1/5
  BW Late September AM Direction/1 -> Multiport Switch1/6
  BW Late September PM Direction/1 -> Multiport Switch1/7
  Space Port July Avg Velocity/1 -> ?
  Space Port Oct Avg Velocity1/1 -> ?
  Space Port Oct Avg Direction/1 -> ?
  Space Port July Avg Direction/1 -> ?
  Jun Avg/1 -> Wind Speed Selector/7
  Jan Avg/1 -> Wind Speed Selector/2
  April Avg/1 -> Wind Speed Selector/5
  March Avg/1 -> Wind Speed Selector/4
  May Avg/1 -> Wind Speed Selector/6
  Feb Avg/1 -> Wind Speed Selector/3
  July Avg/1 -> Wind Speed Selector/8
  Aug Avg/1 -> Wind Speed Selector/9
  Sep Avg/1 -> Wind Speed Selector/10
  Oct Avg/1 -> Wind Speed Selector/11
  Nov Avg/1 -> Wind Speed Selector/12
  Dec Avg/1 -> Wind Speed Selector/13
  Control Input/1 -> Wind Direction Selector/1, Wind Speed Selector/1, Multiport Switch1/1, Multiport Switch/1
  Sep Avg1/1 -> Wind Direction Selector/10
  Jun Avg1/1 -> Wind Direction Selector/7
  March Avg1/1 -> Wind Direction Selector/4
  Oct Avg1/1 -> Wind Direction Selector/11
  July Avg1/1 -> Wind Direction Selector/8
  April Avg1/1 -> Wind Direction Selector/5
  Feb Avg1/1 -> Wind Direction Selector/3
  Jan Avg1/1 -> Wind Direction Selector/2
  Dec Avg1/1 -> Wind Direction Selector/13
  Aug Avg1/1 -> Wind Direction Selector/9
  May Avg1/1 -> Wind Direction Selector/6
  Nov Avg1/1 -> Wind Direction Selector/12
  Wind Speed Selector/1 -> Product/1, Product1/1
  Wind Direction Selector/1 -> Angle Conversion/1
  Wind Random Input X/1 -> Product1/3
  Wind Random Input Y/1 -> Product/3

== system vehicle_simulation/Simulation/RLV/Global Reference Frame/Rocket Frame to Earth Frame ==
  vector X : Inport
  vector Y : Inport  Port=2
  Angle X : Inport  Port=3
  Angle Y : Inport  Port=4
  Angle Z : Inport  Port=5
  vector Z : Inport  Port=6
  Euler Transform for X : MATLAB Function  TreatAsAtomicUnit=on
  Euler Transform for Y : MATLAB Function  TreatAsAtomicUnit=on
  Euler Transform for Z : MATLAB Function  TreatAsAtomicUnit=on
  Earth Frame X(Upward) : Outport  VectorParamsAs1DForOutWhenUnconnected=off
  Earth Frame Y : Outport  Port=2  VectorParamsAs1DForOutWhenUnconnected=off
  Earth Frame Z : Outport  Port=3  VectorParamsAs1DForOutWhenUnconnected=off
  wires:
  vector X/1 -> Euler Transform for Z/1(Fx), Euler Transform for Y/1(Fx), Euler Transform for X/1(Fx)
  vector Y/1 -> Euler Transform for X/2(Fy), Euler Transform for Z/2(Fy), Euler Transform for Y/2(Fy)
  Angle X/1 -> Euler Transform for X/6(AngX), Euler Transform for Z/4(AngX), Euler Transform for Y/4(AngX)
  Angle Y/1 -> Euler Transform for Y/5(AngY), Euler Transform for X/4(AngY), Euler Transform for Z/5(AngY)
  Angle Z/1 -> Euler Transform for Y/6(AngZ), Euler Transform for X/5(AngZ)
  Euler Transform for X/1(y) -> Earth Frame X(Upward)/1
  Euler Transform for Y/1(y) -> Earth Frame Y/1
  Euler Transform for Z/1(y) -> Earth Frame Z/1
  vector Z/1 -> Euler Transform for Z/3(Fz), Euler Transform for Y/3(Fz), Euler Transform for X/3(Fz)

== system vehicle_simulation/Simulation/RLV/Rocket Moments/Simulink Function ==
  f : TriggerPort  TriggerType=function-call  IsSimulinkFunction=on  FunctionName=f  FunctionVisibility=scoped  VariantControl=(inherit)
  Divide : Product  Inputs=*/
  Product : Product
  Product1 : Product
  Subtract : Sum  Inputs=+-
  Subtract1 : Sum  Inputs=+-
  u : ArgIn  DisableCoverage=on  ArgumentName=Tp
  u1 : ArgIn  DisableCoverage=on  Port=2  ArgumentName=Iroll
  u2 : ArgIn  DisableCoverage=on  Port=3  ArgumentName=Iyaw
  u3 : ArgIn  DisableCoverage=on  Port=4  ArgumentName=Ipitch
  u4 : ArgIn  DisableCoverage=on  Port=5  ArgumentName=Wroll
  u5 : ArgIn  DisableCoverage=on  Port=6  ArgumentName=Wyaw
  y : ArgOut  DisableCoverage=on  ArgumentName=y
  wires:
  u/1 -> Subtract1/1
  u1/1 -> Subtract/1
  u2/1 -> Subtract/2
  Subtract/1 -> Product/1
  u4/1 -> Product/2
  u5/1 -> Product1/2
  Product/1 -> Product1/1
  u3/1 -> Divide/2
  Product1/1 -> Subtract1/2
  Subtract1/1 -> Divide/1
  Divide/1 -> y/1

== matlab function vehicle_simulation/Simulation/ALP/ALP acceleration Z ==
  data: trig input; y output; ALPmass input; g input; ChuteArea input; V input; rho input; h input
function y = fcn(trig,ALPmass,g,ChuteArea,V,rho, h)
Cd = 1.2;
if trig == 0 && h > 0
    y = 0.5*Cd*ChuteArea*rho*V^2/ALPmass - g;
else
    y = 0;
end

== matlab function vehicle_simulation/Simulation/ALP/ALP acceleration X ==
  data: trig input; y output; ALPmass input; windV input; CrossSection input; V input; rho input
function y = fcn(trig,ALPmass,windV,CrossSection,V,rho)
Cd = 0.5;
if trig == 0
    y = 0.5*Cd*CrossSection*rho*windV*abs(windV)/ALPmass - 0.5*Cd*CrossSection*rho*V*abs(V)/ALPmass;
else
    y = 0;
end

== matlab function vehicle_simulation/Simulation/ALP/ALP acceleration Y ==
  data: trig input; y output; ALPmass input; windV input; CrossSection input; V input; rho input
function y = fcn(trig,ALPmass,windV,CrossSection,V,rho)
Cd = 0.5;
if trig == 0
    y = 0.5*Cd*CrossSection*rho*windV*abs(windV)/ALPmass - 0.5*Cd*CrossSection*rho*V*abs(V)/ALPmass;
else
    y = 0;
end

== matlab function vehicle_simulation/Simulation/RLV/drogue trigger ==
  data: h input; y output; drogue_dply_alt input; trig input; abort input; V input
function y = fcn(h,drogue_dply_alt, trig, abort, V)

if h <= drogue_dply_alt && ((trig == 1 || abort == 1)) && V < 0 
    y = 0;
else
    y = 1;
end

== matlab function vehicle_simulation/Simulation/RLV/main trigger ==
  data: h input; y output; main_dply_alt input; trig input; abort input; V input
function y = fcn(h,main_dply_alt, trig, abort, V)

if h <= main_dply_alt && (trig == 1 || abort == 1) && V < 0 
    y = 0;
else
    y = 1;
end

== matlab function vehicle_simulation/Simulation/ALP/MATLAB Function ==
  data: u input; y output; h input
function y = fcn(u, h)

if h == 0
    y = 0;
else
    y = u;
end

== matlab function vehicle_simulation/Simulation/ALP/MATLAB Function1 ==
  data: u input; y output; h input
function y = fcn(u, h)

if h == 0
    y = 0;
else
    y = u;
end

== matlab function vehicle_simulation/Simulation/ALP/MATLAB Function2 ==
  data: u input; y output; h input
function y = fcn(u, h)

if h == 0
    y = 0;
else
    y = u;
end

== matlab function vehicle_simulation/Simulation/ALP/MATLAB Function3 ==
  data: u input; y output; h input
function y = fcn(u, h)

if h == 0
    y = 0;
else
    y = u;
end

== matlab function vehicle_simulation/Simulation/ALP/MATLAB Function4 ==
  data: u input; y output; h input
function y = fcn(u, h)

if h == 0
    y = 0;
else
    y = u;
end

== matlab function vehicle_simulation/Simulation/RLV/Latitude Conversion1 ==
  data: Re input; y output; Lat input; D input
function y = fcn(Re, Lat, D)
 
y = 360*D/(2*3.14*Re) + Lat;

== matlab function vehicle_simulation/Simulation/RLV/Flight Triggers ==
  data: ignition_trig input; y output; abort_trig input
function y = fcn(ignition_trig,abort_trig)

if ignition_trig == 1 || abort_trig == 1
    y = 0;
else
    y = 1;
end

== matlab function vehicle_simulation/Simulation/RLV/MATLAB Function1 ==
  data: u input; y output; h input
function y = fcn(u, h)

if h == 0
    y = u;
else
    y = 0;
end

== matlab function vehicle_simulation/Simulation/Balloon Dynamics/Drag ==
  data: V input; y output; rho_air input; Cd input; R input
function y = fcn(V, rho_air, Cd, R)

y = 0.5*V*abs(V)*3.14*R^2*rho_air*Cd;

== matlab function vehicle_simulation/Simulation/Balloon Dynamics/Lifting Force ==
  data: rho_air input; y output; Vol input; g input
function y = fcn(rho_air, Vol, g)

y = rho_air*Vol*g;

== matlab function vehicle_simulation/Simulation/Balloon Dynamics/R(V)1 ==
  data: V input; y output
function y = fcn(V)
y = (3*V/(4*3.14))^(1/3);

== matlab function vehicle_simulation/Simulation/ALP/Pitch//Yaw//Roll Sim/Damp Torque Yaw1 ==
  data: rho input; l input; y output; w input; x input
function y = fcn(rho,l,w,x)
Cd = 1;
y = 0.5*rho*Cd*x*l^3*w*abs(w)/4;

== matlab function vehicle_simulation/Simulation/RLV/Rocket Dynamic Mass ==
  data: launch_trig input; y output; Total_Mass input; Prop_Mass input; BurnT input; t input; T input
function y = fcn(launch_trig, Total_Mass, Prop_Mass, BurnT, t, T)

if (launch_trig == 1) && (t-T <= BurnT)
    y = Total_Mass - Prop_Mass/BurnT*(t-T);
elseif (launch_trig == 1) && (t-T > BurnT)
    y = Total_Mass - Prop_Mass;
else
    y = Total_Mass;
end

== matlab function vehicle_simulation/Simulation/Balloon Dynamics/Weight ==
  data: m_t input; y output; g input
function y = fcn(m_t, g)

y = m_t*g;

== matlab function vehicle_simulation/Simulation/Balloon Dynamics/Balloon Volume2 ==
  data: m_g input; Ta input; Pa input; y output
function y = fcn(m_g, Ta, Pa)
y = m_g*2077*Ta/Pa;

== matlab function vehicle_simulation/Simulation/ALP/Pitch//Yaw//Roll Sim/Angular Acceleration Yaw ==
  data: Ty input; Ipitch input; y output; Iroll input; Iyaw input; Wroll input; Wpitch input
function y = fcn(Ty, Ipitch, Iroll, Iyaw, Wroll,Wpitch)

y = (Ty - (Ipitch - Iroll)*Wroll*Wpitch)/Iyaw;

== matlab function vehicle_simulation/Simulation/ALP/Pitch//Yaw//Roll Sim/Damp Torque Pitch ==
  data: rho input; l input; y output; w input; x input
function y = fcn(rho,l,w,x)
Cd = 1;
Gain = 50;
y = 0.5*rho*Cd*x*l^3*w*abs(w)/4*Gain;

== matlab function vehicle_simulation/Simulation/ALP/Pitch//Yaw//Roll Sim/Damp Torque Yaw ==
  data: rho input; l input; y output; w input; x input
function y = fcn(rho,l,w,x)
Cd = 1;
Gain = 50;
y = 0.5*rho*Cd*x*l^3*w*abs(w)/4*Gain;

== matlab function vehicle_simulation/Simulation/ALP/Pitch//Yaw//Roll Sim/Damp Torque Yaw2 ==
  data: theta input; y output
function y = fcn(theta)
Gain = 2;
y = Gain*theta;

== matlab function vehicle_simulation/Simulation/ALP/Pitch//Yaw//Roll Sim/Damp Torque Yaw3 ==
  data: theta input; y output
function y = fcn(theta)
Gain = 2;
y = Gain*theta;

== matlab function vehicle_simulation/Simulation/ALP/Pitch//Yaw//Roll Sim/Damp Torque Yaw4 ==
  data: theta input; y output
function y = fcn(theta)
Gain = 2;
y = Gain*theta;

== matlab function vehicle_simulation/Simulation/RLV/Rocket Thrust ==
  data: launch_trig input; y output; BurnT input; t input; T input; Thrust input
function y = fcn(launch_trig, BurnT, t, T, Thrust)

if (launch_trig == 1) && (t-T <= BurnT)
    y = Thrust;
else
    y = 0;
end

== matlab function vehicle_simulation/Simulation/ALP/Power Systems/Heater ON (BATT) ==
  data: TempBat input; y output; TriggerTemp input
function y = fcn(TempBat, TriggerTemp)

if TempBat < TriggerTemp
    y = 1;
else
    y = 0;
end

== matlab function vehicle_simulation/Simulation/ALP/Pitch//Yaw//Roll Sim/Angular Acceleration Pitch ==
  data: Tp input; y output; Iroll input; Iyaw input; Ipitch input; Wroll input; Wyaw input
function y = fcn(Tp, Iroll, Iyaw, Ipitch, Wroll,Wyaw)

y = (Tp - (Iroll - Iyaw)*Wroll*Wyaw)/Ipitch;

== matlab function vehicle_simulation/Simulation/ALP/Longitude Conversion1 ==
  data: Re input; y output; Long input; D input
function y = fcn(Re, Long, D)
 
y = 360*D/(2*3.14*Re) + Long;

== matlab function vehicle_simulation/Simulation/ALP/Latitude Conversion1 ==
  data: Re input; y output; Lat input; D input
function y = fcn(Re, Lat, D)
 
y = 360*D/(2*3.14*Re) + Lat;

== matlab function vehicle_simulation/Simulation/ALP/Power Systems/Heater ON (BOARD) ==
  data: Temp input; y output; TriggerTemp input
function y = fcn(Temp, TriggerTemp)

if Temp < TriggerTemp
    y = 1;
else
    y = 0;
end

== matlab function vehicle_simulation/Simulation/RLV/Longitude Conversion1 ==
  data: Re input; y output; Long input; D input
function y = fcn(Re, Long, D)
 
y = 360*D/(2*3.14*Re) + Long;

== matlab function vehicle_simulation/Simulation/RLV/Force X ==
  data: y output; CrossSec input; rho input; V input; droque input; main input; trig input; abort input; In input; M input
function y = fcn(CrossSec,rho,V, droque, main, trig, abort, In, M)

Cd_cross = 1.25;
if droque ~= 0 && main ~= 0 && abort == 0
    y = In/M;
elseif trig == 1 && (droque ~= 1 ||  main ~= 1) 
    y = 0.5*rho*V*abs(V)*Cd_cross*CrossSec/M;
else
    y = 0;
end

== matlab function vehicle_simulation/Simulation/RLV/Force Z ==
  data: y output; CrossSec input; rho input; V input; droque input; main input; trig input; abort input; In input; M input
function y = fcn(CrossSec,rho,V, droque, main, trig, abort, In, M)

Cd_cross = 1.25;
if droque ~= 0 && main ~= 0 && abort == 0
    y = In/M;
elseif trig == 1 && (droque ~= 1 ||  main ~= 1) 
    y = 0.5*rho*V*abs(V)*Cd_cross*CrossSec/M;
else
    y = 0;
end

== matlab function vehicle_simulation/Simulation/RLV/Force Y (alt) ==
  data: Droque input; y output; Main input; CrossSec input; rho input; V input; droque input; main input; trig input; abort input; g input; In input; M input
function y = fcn(Droque,Main, CrossSec,rho,V, droque, main, trig, abort,g,In, M)
Cd_rocket = 0.5;
Cd_para = 1.25;
if trig == 1 && droque ~= 0 && main ~= 0 && abort == 0
    y = In/M-g;
elseif (trig == 1 && droque ~= 1 && main ~= 0) || abort == 1
    y = 0.5*rho*V^2*(Cd_rocket*CrossSec+Cd_para*Droque)/M-g;
elseif (trig == 1 && droque ~= 1 && main ~= 1) || abort == 1
    y = 0.5*rho*V^2*(Cd_rocket*CrossSec+Cd_para*Main)/M-g;
else
    y = 0;
end

== matlab function vehicle_simulation/Simulation/RLV/Global Reference Frame/Rocket Frame to Earth Frame/Euler Transform for X ==
  data: Fx input; y output; Fy input; Fz input; AngY input; AngZ input; AngX input
function y = fcn(Fx, Fy, Fz, AngY, AngZ, AngX)
%#codegen

y = Fx*(cos(AngY)*cos(AngZ)) + Fy*(sin(AngX)*sin(AngY)*cos(AngZ)-cos(AngX)*sin(AngZ)) + Fz*(sin(AngX)*sin(AngZ)+cos(AngX)*sin(AngY)*cos(AngZ));

== matlab function vehicle_simulation/Simulation/RLV/Global Reference Frame/Rocket Frame to Earth Frame/Euler Transform for Y ==
  data: Fx input; y output; Fy input; Fz input; AngX input; AngY input; AngZ input
function y = fcn(Fx, Fy, Fz, AngX, AngY, AngZ)
%#codegen

y = Fx*(cos(AngY))*sin(AngZ)+Fy*(cos(AngX)*cos(AngZ)+sin(AngX)*sin(AngY)*sin(AngZ)) + Fz*(cos(AngX)*sin(AngY)*sin(AngZ)-sin(AngX)*cos(AngZ));

== matlab function vehicle_simulation/Simulation/RLV/Global Reference Frame/Rocket Frame to Earth Frame/Euler Transform for Z ==
  data: Fx input; y output; Fy input; Fz input; AngX input; AngY input
function y = fcn(Fx, Fy, Fz, AngX, AngY)
%#codegen

y = -Fx*sin(AngY) + Fy*(sin(AngX)*cos(AngY)) + Fz*(cos(AngX)*sin(AngY));

== matlab function vehicle_simulation/Simulation/Flight Triggers ==
  data: ignition_trig input; y output; abort_trig input
function y = fcn(ignition_trig,abort_trig)

if ignition_trig == 1 || abort_trig == 1
    y = 0;
else
    y = 1;
end

== matlab function vehicle_simulation/Simulation/RLV/Rocket Moments/Angular Acceleration Pitch ==
  data: Tp input; y output; Iroll input; Iyaw input; Ipitch input; Wroll input; Wyaw input
function y = fcn(Tp, Iroll, Iyaw, Ipitch, Wroll,Wyaw)

y = (Tp - (Iroll - Iyaw)*Wroll*Wyaw)/Ipitch;

== matlab function vehicle_simulation/Simulation/RLV/Rocket Moments/Angular Acceleration Yaw ==
  data: Ty input; Ipitch input; y output; Iroll input; Iyaw input; Wroll input; Wpitch input
function y = fcn(Ty, Ipitch, Iroll, Iyaw, Wroll,Wpitch)

y = (Ty - (Ipitch - Iroll)*Wroll*Wpitch)/Iyaw;

== matlab function vehicle_simulation/Simulation/RLV/MATLAB Function2 ==
  data: i input; y output; j input; k input
function y = fcn(i,j,k)

y = (i^2+j^2+k^2)^0.5;

== matlab function vehicle_simulation/Simulation/RLV/Force Pitch ==
  data: theta input; y output; Cd input; CrossSec input; rho input; V input; droque input; main input; trig input; abort input
function y = fcn(theta, Cd, CrossSec,rho,V, droque, main, trig, abort)

if trig == 1 && droque ~= 0 && main ~= 0 && abort == 0
    y = 0.5*rho*CrossSec*V*abs(V)*Cd*sin(theta);
else
    y = 0;
end

== matlab function vehicle_simulation/Simulation/RLV/Force Yaw ==
  data: theta input; y output; Cd input; CrossSec input; rho input; V input; droque input; main input; trig input; abort input
function y = fcn(theta, Cd, CrossSec,rho,V, droque, main, trig, abort)

if trig == 1 && droque ~= 0 && main ~= 0 && abort == 0
    y = 0.5*rho*CrossSec*V*abs(V)*Cd*sin(theta);
else
    y = 0;
end

== matlab function vehicle_simulation/Simulation/Balloon Dynamics/balloon acceleration X ==
  data: Cd input; y output; V input; VwindX input; m input; air_rho input; Vol input
function y = fcn(Cd,V,VwindX,m,air_rho,Vol)

Ac = pi*(3/(4*pi)*Vol)^2/3;
F_wind = 0.5*Cd*VwindX*abs(VwindX)*air_rho*Ac;
F_drag = 0.5*air_rho*V*abs(V)*Ac*Cd;
y= F_wind/m - F_drag/m;

== matlab function vehicle_simulation/Simulation/Balloon Dynamics/balloon acceleration Y ==
  data: Cd input; y output; V input; VwindX input; m input; air_rho input; Vol input
function y = fcn(Cd,V,VwindX,m,air_rho,Vol)

Ac = pi*(3/(4*pi)*Vol)^2/3;
F_wind = 0.5*Cd*VwindX*abs(VwindX)*air_rho*Ac;
F_drag = 0.5*air_rho*V*abs(V)*Ac*Cd;
y= F_wind/m - F_drag/m;

== matlab function vehicle_simulation/Simulation/Mass of Balloon ==
  data: thickness input; y output; Area input; density input
function y = fcn(thickness,Area,density)

y = thickness*Area*density;

== matlab function vehicle_simulation/Simulation/RLV/Force Axial ==
  data: Thrust input; y output; Cd input; CrossSec input; rho input; V input; droque input; main input; trig input; abort input
function y = fcn(Thrust, Cd, CrossSec,rho,V, droque, main, trig, abort)
 
if trig == 1 && droque ~= 0 && main ~= 0 && abort == 0
    y = Thrust - 0.5*rho*CrossSec*V^2*Cd;
else
    y = 0;
end
